simulink model "LQG_Sim"  (R2018a)
settings: Solver=VariableStepAuto  StartTime=0.0  StopTime=t_final  RelTol=1e-3
values from neighbouring files (symbols this model uses):
  A = [0                     1                           0              0 ... (first row only)    [TuBesKL_Part1.m]    (also in TuBesKL_Part2.m = [0                     1                           0        ; TuBesKL_Part3.m = [0                     1                           0        )
  B = [0 ; 2*km*(Ip*+mp*l^2-mp*l*r)/Ri*r*A1 ; 0 ;(2*km)*(mp*l-r*B1)/Ri*r*A1]    [TuBesKL_Part1.m]    (also in TuBesKL_Part2.m = [0 ; 2*km*(Ip*+mp*l^2-mp*l*r)/Ri*r*A1 ; 0 ; (2*km)*(mp*l-r*B; TuBesKL_Part3.m = [0 ; 2*km*(Ip*+mp*l^2-mp*l*r)/Ri*r*A1 ; 0 ; (2*km)*(mp*l-r*B)
  C = [1 0 0 0;0 0 1 0]    [TuBesKL_Part1.m]    (also in TuBesKL_Part2.m; TuBesKL_Part3.m = [1 0 0 0])
  K = lqr(A,B,Q,R)    [TuBesKL_Part3.m]
  Kf = (lqr(A',C(1,:)',Wd,Wn))'    [TuBesKL_Part2.m]    (also in TuBesKL_Part3.m = (lqr(A',C',Wd,Wn))')
settings Model: Creator=user  LastModifiedBy=Haris Widiarta

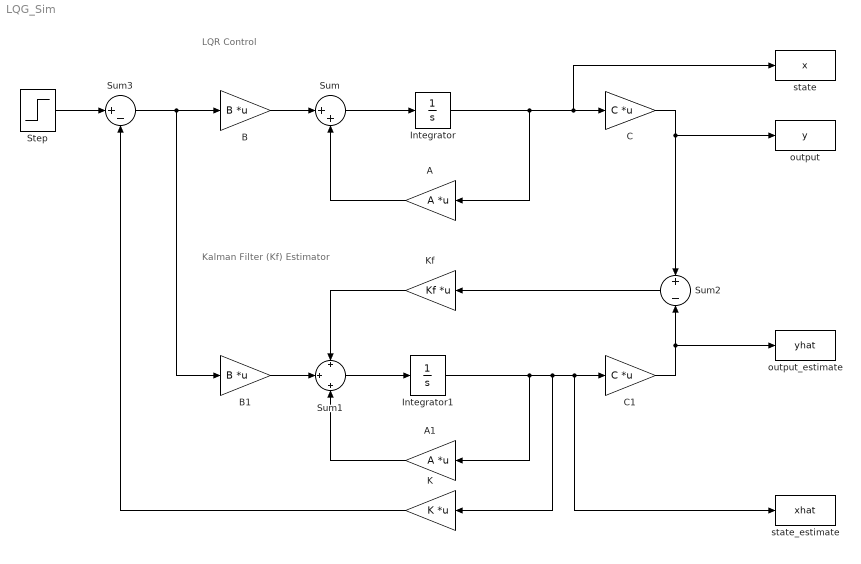
== system LQG_Sim ==
  note: Kalman Filter (Kf) Estimator
  note: LQR Control
  A : Gain  Gain=A  Multiplication=Matrix(K*u)
  A1 : Gain  Gain=A  Multiplication=Matrix(K*u)
  B : Gain  Gain=B  Multiplication=Matrix(K*u)
  B1 : Gain  Gain=B  Multiplication=Matrix(K*u)
  C : Gain  Gain=C  Multiplication=Matrix(K*u)
  C1 : Gain  Gain=C  Multiplication=Matrix(K*u)
  Integrator : Integrator  InitialCondition=[5;10;15;20]
  Integrator1 : Integrator  InitialCondition=[0;0;0;0]
  K : Gain  Gain=K  Multiplication=Matrix(K*u)
  Kf : Gain  Gain=Kf  Multiplication=Matrix(K*u)
  Step : Step  SampleTime=0
  Sum : Sum  Inputs=|++
  Sum1 : Sum  Inputs=+|+|+
  Sum2 : Sum  Inputs=+|-
  Sum3 : Sum  Inputs=|+-
  output : ToWorkspace  VariableName=y  SaveFormat=Structure With Time  SampleTime=-1
  output_estimate : ToWorkspace  VariableName=yhat  SaveFormat=Structure With Time  SampleTime=-1
  state : ToWorkspace  VariableName=x  SaveFormat=Structure With Time  SampleTime=-1
  state_estimate : ToWorkspace  VariableName=xhat  SaveFormat=Structure With Time  SampleTime=-1
  wires:
  Sum/1 -> Integrator/1
  Integrator/1 -> A/1, state/1, C/1
  Integrator1/1 -> A1/1, K/1, state_estimate/1, C1/1
  Sum1/1 -> Integrator1/1
  C1/1 -> output_estimate/1, Sum2/2
  Sum2/1 -> Kf/1
  A1/1 -> Sum1/3
  B1/1 -> Sum1/2
  Kf/1 -> Sum1/1
  A/1 -> Sum/2
  B/1 -> Sum/1
  C/1 -> Sum2/1, output/1
  K/1 -> Sum3/2
  Sum3/1 -> B/1, B1/1
  Step/1 -> Sum3/1
